simulink model "DC_gearmotor_plus_resonant_load"  (R2024b)
settings: Solver=VariableStepAuto  StartTime=0.0  StopTime=10.0  RelTol=1e-3
undefined symbols (not defined in the file): gbox, mld, mot, rads2rpm, sens
settings Model: Creator=Enrico  LastModifiedBy=Enrico

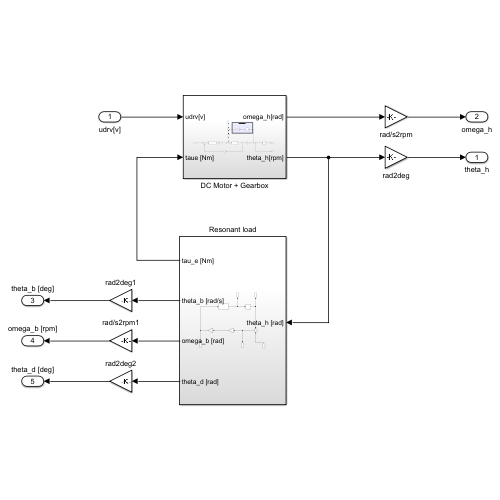
[thumbnail: Simulink's stored preview of the top-level diagram]
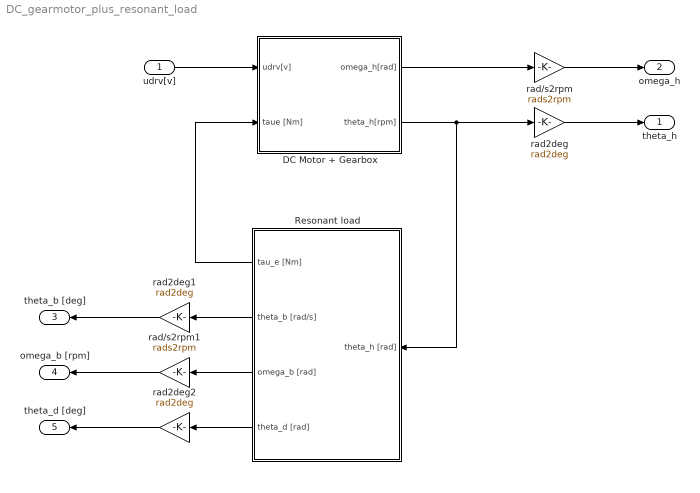
== system DC_gearmotor_plus_resonant_load ==
  udrv[v] : Inport
  DC Motor + Gearbox : Subsystem
  Resonant load : Subsystem
  rad/s2rpm : Gain  Gain=rads2rpm
  rad/s2rpm1 : Gain  Gain=rads2rpm
  rad2deg : Gain  Gain=rad2deg
  rad2deg1 : Gain  Gain=rad2deg
  rad2deg2 : Gain  Gain=rad2deg
  theta_h : Outport
  omega_h : Outport  Port=2
  theta_b [deg] : Outport  Port=3
  omega_b [rpm] : Outport  Port=4
  theta_d [deg] : Outport  Port=5
  wires:
  Resonant load/1(tau_e [Nm]) -> DC Motor + Gearbox/2(taue [Nm])
  Resonant load/2(theta_b [rad/s]) -> rad2deg1/1
  Resonant load/3(omega_b [rad]) -> rad/s2rpm1/1
  DC Motor + Gearbox/2(theta_h[rpm]) -> rad2deg/1, Resonant load/1(theta_h [rad])
  rad/s2rpm1/1 -> omega_b [rpm]/1
  DC Motor + Gearbox/1(omega_h[rad]) -> rad/s2rpm/1
  rad2deg1/1 -> theta_b [deg]/1
  rad2deg/1 -> theta_h/1
  udrv[v]/1 -> DC Motor + Gearbox/1(udrv[v])
  Resonant load/4(theta_d [rad]) -> rad2deg2/1
  rad/s2rpm/1 -> omega_h/1
  rad2deg2/1 -> theta_d [deg]/1

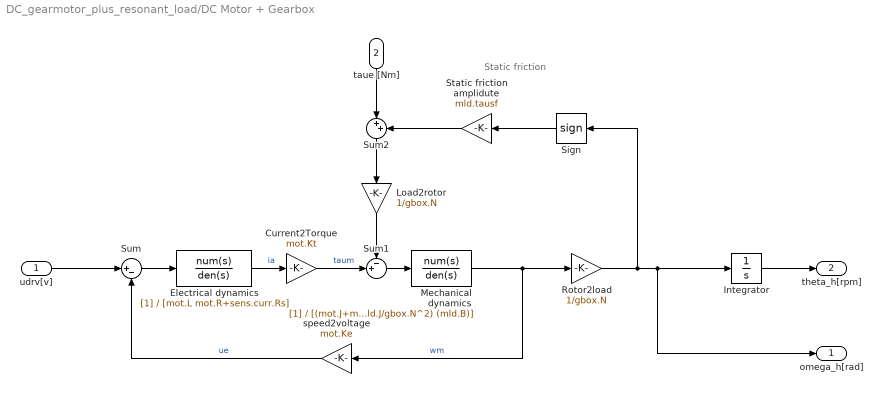
== system DC_gearmotor_plus_resonant_load/DC Motor + Gearbox ==
  note: Static friction
  udrv[v] : Inport
  taue [Nm] : Inport  Port=2
  " Sign" : Signum  ZeroCross=off
  Current2Torque : Gain  Gain=mot.Kt
  Electrical dynamics : TransferFcn  Denominator=[mot.L mot.R+sens.curr.Rs]
  Integrator : Integrator
  Load2rotor : Gain  Gain=1/gbox.N
  Mechanical dynamics : TransferFcn  Denominator=[(mot.J+mld.J/gbox.N^2) (mld.B)]
  Rotor2load : Gain  Gain=1/gbox.N
  Static friction amplidute : Gain  Gain=mld.tausf
  Sum : Sum  Inputs=|+-
  Sum1 : Sum  Inputs=-+|
  Sum2 : Sum  Inputs=|++
  speed2voltage : Gain  Gain=mot.Ke
  omega_h[rad] : Outport
  theta_h[rpm] : Outport  Port=2
  wires:
  udrv[v]/1 -> Sum/1
  Sum/1 -> Electrical dynamics/1
  Electrical dynamics/1 -> Current2Torque/1  "ia"
  Current2Torque/1 -> Sum1/2  "taum"
  Load2rotor/1 -> Sum1/1
  " Sign"/1 -> Static friction amplidute/1
  Sum1/1 -> Mechanical dynamics/1
  Mechanical dynamics/1 -> speed2voltage/1, Rotor2load/1  "wm"
  speed2voltage/1 -> Sum/2  "ue"
  Rotor2load/1 -> " Sign"/1, omega_h[rad]/1, Integrator/1
  Sum2/1 -> Load2rotor/1
  Static friction amplidute/1 -> Sum2/2
  taue [Nm]/1 -> Sum2/1
  Integrator/1 -> theta_h[rpm]/1

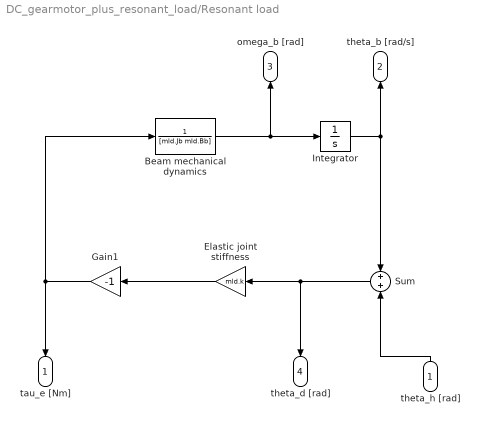
== system DC_gearmotor_plus_resonant_load/Resonant load ==
  theta_h [rad] : Inport
  Beam mechanical dynamics : TransferFcn  Denominator=[mld.Jb mld.Bb]
  Elastic joint stiffness : Gain  Gain=mld.k
  Gain1 : Gain  Gain=-1
  Integrator : Integrator
  Sum : Sum  Inputs=+|+
  tau_e [Nm] : Outport
  theta_b [rad/s] : Outport  Port=2
  omega_b [rad] : Outport  Port=3
  theta_d [rad] : Outport  Port=4
  wires:
  theta_h [rad]/1 -> Sum/2
  Gain1/1 -> tau_e [Nm]/1, Beam mechanical dynamics/1
  Sum/1 -> Elastic joint stiffness/1, theta_d [rad]/1
  Integrator/1 -> theta_b [rad/s]/1, Sum/1
  Elastic joint stiffness/1 -> Gain1/1
  Beam mechanical dynamics/1 -> omega_b [rad]/1, Integrator/1
